simulink model "Position_errors 2"  (R2019a)
settings: Solver=VariableStepAuto  StartTime=0.0  StopTime=10.0  RelTol=1e-3
undefined symbols (not defined in the file): error_margin, Ts
settings Model: Creator=mrblissfulgrin  LastModifiedBy=mrblissfulgrin

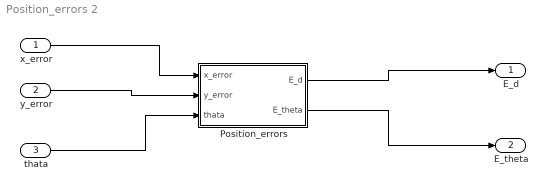
== system Position_errors 2 ==
  x_error : Inport
  y_error : Inport  Port=2
  thata : Inport  Port=3
  Position_errors : Subsystem
  E_d : Outport
  E_theta : Outport  Port=2
  wires:
  x_error/1 -> Position_errors/1(x_error)
  y_error/1 -> Position_errors/2(y_error)
  thata/1 -> Position_errors/3(thata)
  Position_errors/1(E_d) -> E_d/1
  Position_errors/2(E_theta) -> E_theta/1

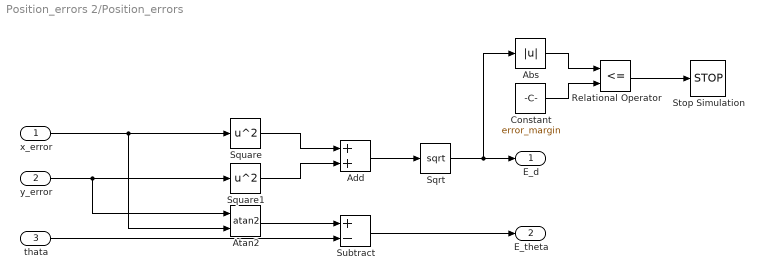
== system Position_errors 2/Position_errors ==
  x_error : Inport  SampleTime=Ts
  y_error : Inport  Port=2  SampleTime=Ts
  thata : Inport  Port=3  SampleTime=Ts
  Abs : Abs
  Add : Sum
  Atan2 : Trigonometry  Operator=atan2
  Constant : Constant  Value=error_margin
  Relational Operator : RelationalOperator  Operator=<=  OutDataTypeStr=boolean  RndMeth=Simplest
  Sqrt : Sqrt  SaturateOnIntegerOverflow=on
  Square : Math  Operator=square  SaturateOnIntegerOverflow=on
  Square1 : Math  Operator=square  SaturateOnIntegerOverflow=on
  Stop Simulation : Stop
  Subtract : Sum  Inputs=+-
  E_d : Outport  SampleTime=Ts
  E_theta : Outport  Port=2  SampleTime=Ts
  wires:
  Square/1 -> Add/1
  Atan2/1 -> Subtract/1
  Sqrt/1 -> E_d/1, Abs/1
  y_error/1 -> Square1/1, Atan2/1
  Add/1 -> Sqrt/1
  Square1/1 -> Add/2
  thata/1 -> Subtract/2
  x_error/1 -> Square/1, Atan2/2
  Subtract/1 -> E_theta/1
  Abs/1 -> Relational Operator/1
  Constant/1 -> Relational Operator/2
  Relational Operator/1 -> Stop Simulation/1
